simulink model "Qdesign_simulation"  (R2018b)
settings: Solver=VariableStepAuto  StartTime=0.0  StopTime=10.0  RelTol=1e-3
values from neighbouring files (symbols this model uses):
  lower_lim = -2.5    [part2-viral.m]    (also in part2.m; part2_Nathan.m; qdesign-viral.m)
  ss1_den = [1.8 4.5 1]    [part2-viral.m]    (also in part2.m; part2_Nathan.m; qdesign-viral.m)
  ss1_num = 0.1    [part2-viral.m]    (also in part2.m; part2_Nathan.m; qdesign-viral.m)
  upper_lim = 2.5    [part2-viral.m]    (also in part2.m; part2_Nathan.m; qdesign-viral.m)
libraries: cstblocks x2
settings Model: Creator=viral  LastModifiedBy=viral

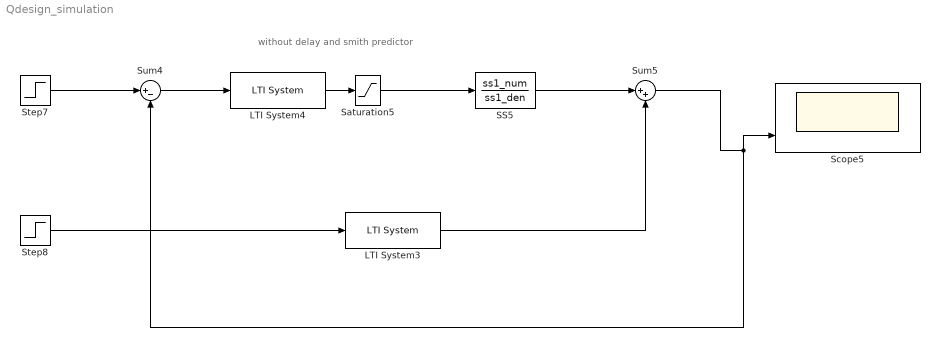
== system Qdesign_simulation ==
  note: without delay and smith predictor
  LTI System3 : cstblocks/LTI System  sys=g2  IC=[]
  LTI System4 : cstblocks/LTI System  sys=C  IC=[]
  SS5 : TransferFcn  Numerator=ss1_num  Denominator=ss1_den
  Saturation5 : Saturate  UpperLimit=upper_lim  LowerLimit=lower_lim
  Scope5 : Scope  NumInputPorts=2
  Step7 : Step  Time=5  SampleTime=0
  Step8 : Step  Time=25  After=0.1  SampleTime=0
  Sum4 : Sum  Inputs=|+-
  Sum5 : Sum  Inputs=|++
  wires:
  Sum4/1 -> LTI System4/1
  Step7/1 -> Sum4/1
  Step8/1 -> LTI System3/1
  Sum5/1 -> Sum4/2, Scope5/2
  LTI System3/1 -> Sum5/2
  LTI System4/1 -> Saturation5/1
  Saturation5/1 -> SS5/1
  SS5/1 -> Sum5/1
